simulink model "link3manip"  (R2018b)
settings: Solver=FixedStepAuto  StartTime=0.0  StopTime=inf  RelTol=1e-3  EnableMultiTasking=on
libraries: c2000scilib x3, demo_controls x1
settings Model: Creator=aancelle  LastModifiedBy=Ali
settings DataIOCC: LimitDataPoints=on  SaveFormat=Array  SignalLoggingSaveFormat=ModelDataLogs
settings OptimizationCC: BlockReduction=off  LifeSpan=1
settings DebuggingCC: UnderspecifiedInitializationDetection=Classic  MergeDetectMultiDrivingBlocksExec=none  SolverPrmCheckMsg=warning  AllowSymbolicDim=off  SFUnexpectedBacktrackingDiag=warning  SFNoUnconditionalDefaultTransitionDiag=warning  SFExecutionAtInitializationDiag=none
settings HardwareCC: ProdBitPerPointer=32  ProdBitPerSizeT=32  ProdBitPerPtrDiffT=32  ProdLargestAtomicFloat=None  ProdIntDivRoundTo=Undefined  ProdEndianess=Unspecified  ProdWordSize=32  ProdHWDeviceType=32-bit Generic
settings ModelReferenceCC: PropagateSignalLabelsOutOfModel=off
settings SFSimCC: SimUseLocalCustomCode=off  MATLABDynamicMemAlloc=off
settings RTWCC: SystemTargetFile=ert.tlc  TemplateMakefile=ert_default_tmf  Description=Real-Time Workshop Embedded Coder  GenerateReport=on  RTWUseLocalCustomCode=off  IncludeHyperlinkInReport=on  LaunchReport=on  GenerateTraceInfo=on  GenerateTraceReport=on  GenerateTraceReportSl=on  GenerateTraceReportSf=on  GenerateTraceReportEml=on
settings CodeAppCC: IgnoreCustomStorageClasses=off  StateflowObjectComments=on  InternalIdentifier=Classic
settings ERTTargetCC: MultiwordLength=2048  GenerateSampleERTMain=on  ERTCustomFileTemplate=example_file_process.tlc  ConvertIfToSwitch=off  SuppressUnreachableDefaultCases=off
settings ConfigComp: CovMetricSettings=dw  CovHtmlReporting=on  CovSaveCumulativeToWorkspaceVar=on  CovSaveSingleToWorkspaceVar=on  CovExternalEMLEnable=off

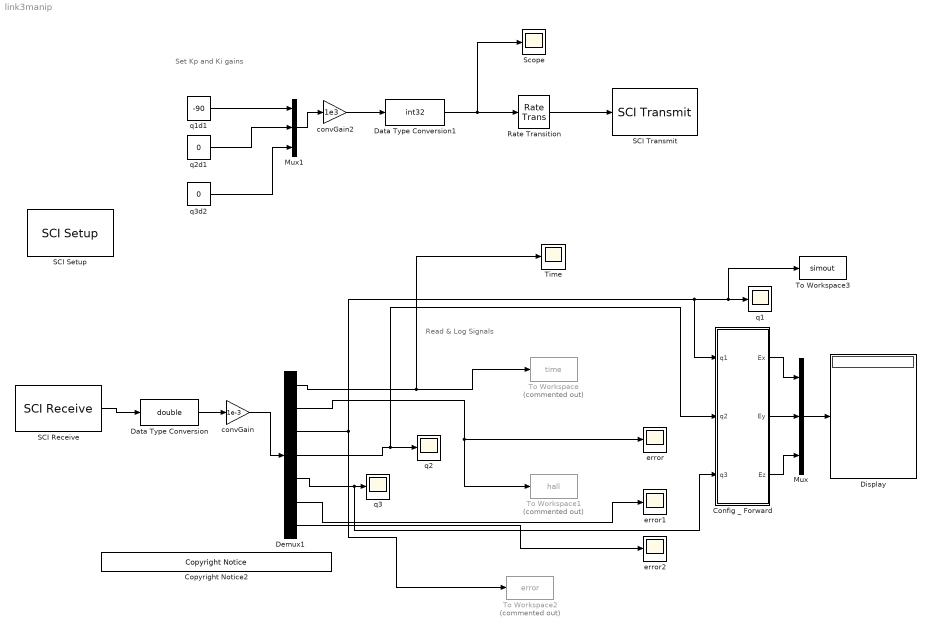
== system link3manip ==
  note: Read & Log Signals
  note: Set Kp and Ki gains
  Config _ Forward : MATLAB Function  TreatAsAtomicUnit=on
  Copyright Notice2 : demo_controls/Copyright Notice  year=2014  prod=tic2000
  Data Type Conversion : DataTypeConversion  OutDataTypeStr=double  ConvertRealWorld=Stored Integer (SI)
  Data Type Conversion1 : DataTypeConversion  OutDataTypeStr=int32  ConvertRealWorld=Stored Integer (SI)
  Demux1 : Demux  Outputs=7
  Display : Display
  Mux : Mux  Inputs=3
  Mux1 : Mux  Inputs=3
  Rate Transition : RateTransition  OutPortSampleTime=0.05
  SCI Receive : c2000scilib/SCI Receive  module=COM 2  dataHead='S'  dataTail='E'  dataType=int32  dataDim=7  initValue=0  errOption=Output the last received value  errValue=0  sampleTime=0.02  outputStatus=off
      settings: SourceProductName=MATLAB Coder  SourceProductBaseCode=ME
  SCI Setup : c2000scilib/SCI Setup  Priority=-99  commModeA=raw data  baudRateA=115200  charLenA=8  stopBitA=1  parityA=none  timeoutA=1.0  commModeB=raw data  baudRateB=115200  charLenB=8  stopBitB=1  parityB=none  timeoutB=1.0  commModeC=raw data  baudRateC=115200  charLenC=8  stopBitC=1  parityC=none  timeoutC=1.0  commModeD=raw data  baudRateD=115200  charLenD=8  stopBitD=1  parityD=none  timeoutD=1.0
      settings: SourceProductName=MATLAB Coder  SourceProductBaseCode=ME
  SCI Transmit : c2000scilib/SCI Transmit  module=COM 2  header='S'  tail='E'
      settings: SourceProductName=MATLAB Coder  SourceProductBaseCode=ME
  Scope : Scope
  Time : Scope
  To Workspace : ToWorkspace  Commented=on  VariableName=time  SaveFormat=Timeseries  SampleTime=-1
  To Workspace1 : ToWorkspace  Commented=on  VariableName=hall  SaveFormat=Timeseries  SampleTime=-1
  To Workspace2 : ToWorkspace  Commented=on  VariableName=error  SaveFormat=Timeseries  SampleTime=-1
  To Workspace3 : ToWorkspace  VariableName=simout  SampleTime=-1
      settings: Save2DSignal=2-D array (concatenate along first dimension)
  convGain : Gain  Gain=1e-3
  convGain2 : Gain  Gain=1e3
  error : Scope
  error1 : Scope
  error2 : Scope
  q1 : Scope
  q1d1 : Constant  Value=-90
  q2 : Scope
  q2d1 : Constant  Value=0
  q3 : Scope
  q3d2 : Constant  Value=0
  wires:
  SCI Receive/1 -> Data Type Conversion/1
  Data Type Conversion/1 -> convGain/1
  Demux1/1 -> To Workspace/1, Time/1
  Mux1/1 -> convGain2/1
  convGain/1 -> Demux1/1
  Data Type Conversion1/1 -> Scope/1, Rate Transition/1
  Rate Transition/1 -> SCI Transmit/1
  convGain2/1 -> Data Type Conversion1/1
  Demux1/2 -> To Workspace1/1, error/1
  Demux1/3 -> To Workspace2/1, Config _ Forward/1(q1), To Workspace3/1, q1/1
  Demux1/4 -> Config _ Forward/2(q2), q2/1
  Demux1/5 -> Config _ Forward/3(q3), q3/1
  Demux1/6 -> error1/1
  Demux1/7 -> error2/1
  Config _ Forward/3(Ez) -> Mux/3
  Config _ Forward/2(Ey) -> Mux/2
  Config _ Forward/1(Ex) -> Mux/1
  Mux/1 -> Display/1
  q2d1/1 -> Mux1/2
  q3d2/1 -> Mux1/3
  q1d1/1 -> Mux1/1

== matlab function link3manip/Config _ Forward ==
  data: Ex output; Ey output; q1 input; q2 input; q3 input; Ez output
function [Ex, Ey, Ez]= fcn(q1, q2, q3)

%link lengths
l1 = 105.8;
l2 = 98.7459;
l3 = 140.2516;

%Transformation matrices btw consecutive bodies
H_1_0 = [cos(q1) 0 sin(q1) 0; sin(q1) 0 -cos(q1) 0; 0 1 0 l1; 0 0 0 1];
H_2_1 = [cos(q2) -sin(q2) 0 l2*cos(q2); sin(q2) cos(q2) 0 l2*sin(q2); 0 0 1 0; 0 0 0 1];
H_3_2 = [cos(q3) 0 sin(q3) l3*cos(q3); sin(q3) 0 -cosd(q3) l3*sin(q3); 0 1 0 0; 0 0 0 1];

H_3_0 = H_1_0 * H_2_1 * H_3_2;

%End effector positions
Ex = H_3_0(1,4);
Ey = H_3_0(2,4);
Ez = H_3_0(3,4);
